simulink model "ultrasonic_sensor"  (R2019a)
settings: Solver=FixedStepAuto  StartTime=0.0  StopTime=inf  RelTol=1e-3  EnableMultiTasking=on
libraries: embdlinuxlib x4, dspswit3 x1
settings Model: SimulationMode=external  Creator=wojna  LastModifiedBy=wojna
settings SolverCC: PositivePriorityOrder=on
settings OptimizationCC: EnhancedBackFolding=on  PassReuseOutputArgsAs=Individual arguments  MaxStackSize=64  OptimizeBlockOrder=speed  DifferentSizesBufferReuse=on  OptimizationCustomize=off
settings DebuggingCC: ParameterTunabilityLossMsg=error
settings HardwareCC: ProdBitPerPointer=32  ProdBitPerSizeT=32  ProdBitPerPtrDiffT=32  ProdLargestAtomicInteger=Long  ProdLargestAtomicFloat=Double  ProdWordSize=32  ProdLongLongMode=on  ProdHWDeviceType=ARM Compatible->ARM Cortex  UseEmbeddedCoderFeatures=off  UseSimulinkCoderFeatures=off
settings SFSimCC: MATLABDynamicMemAlloc=off
settings RTWCC: SystemTargetFile=ert.tlc  HardwareBoard=Raspberry Pi  TLCOptions="-aInlineSetEventsForThisBaseRateFcn=TLC_FALSE -aSuppressMultiTaskScheduler=TLC_FALSE  -aRateBasedStepFcn=0"  TemplateMakefile=ert_default_tmf  RTWVerbose=off  Toolchain=GNU GCC Raspberry Pi  BuildConfiguration=Faster Runs  IncludeHyperlinkInReport=on
settings CodeAppCC: ForceParamTrailComments=on  OperatorAnnotations=on  SimulinkDataObjDesc=on  SFDataObjDesc=on  MangleLength=10  InsertBlockDesc=on
settings ERTTargetCC: SupportNonInlinedSFcns=on  SupportVariableSizeSignals=on  ExtMode=on  ExtModeTransport=2  ExtModeStaticAlloc=on  ExtModeMexFile=ext_xcp  ExtModeMexArgs='192.168.0.101' 0 17725  ExtModeIntrfLevel=Level2 - Open  ERTSrcFileBannerTemplate=codertarget_code_template.cgt  ERTHdrFileBannerTemplate=codertarget_code_template.cgt  ERTDataSrcFileTemplate=codertarget_code_template.cgt  ERTDataHdrFileTemplate=codertarget_code_template.cgt

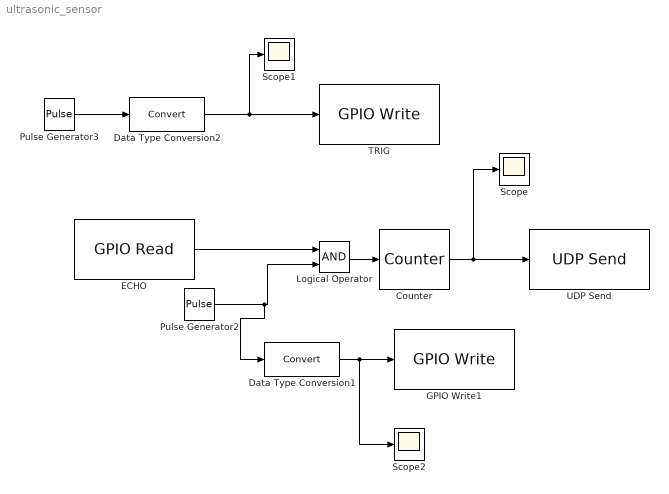
== system ultrasonic_sensor ==
  Counter : dspswit3/Counter  Direction=Up  CountEvent=Rising edge  CounterSize=8 bits  MaxCount=255  InitialCount=0  Output=Count  HitValue=32  ResetInput=off  SamplesPerFrame=1  Ts=1  CntDtype=double  HitDtype=Logical
  Data Type Conversion1 : DataTypeConversion
  Data Type Conversion2 : DataTypeConversion
  ECHO : embdlinuxlib/GPIO Read  board=Pi 3 Model B+  gpio=23  internalResistor=Off  sampleTime=2.5e-05  direction=Input  blockPlatform=Raspberry Pi
      settings: SourceProductName=Simulink Coder Support Package for BeagleBone Blue Hardware  SourceProductBaseCode=SC_BEAGLEBONE_BLUE
  GPIO Write1 : embdlinuxlib/GPIO Write  board=Pi 3 Model B+  gpio=24  direction=Output  blockPlatform=Raspberry Pi
      settings: SourceProductName=Simulink Coder Support Package for BeagleBone Blue Hardware  SourceProductBaseCode=SC_BEAGLEBONE_BLUE
  Logical Operator : Logic  AllPortsSameDT=off  OutDataTypeStr=boolean
  Pulse Generator2 : DiscretePulseGenerator  PulseType=Time based  Amplitude=3  Period=0.00005  PulseWidth=50
  Pulse Generator3 : DiscretePulseGenerator  PulseType=Time based  Amplitude=3  Period=0.1  PulseWidth=0.01
  Scope : Scope
  Scope1 : Scope
  Scope2 : Scope
  TRIG : embdlinuxlib/GPIO Write  board=Pi 3 Model B+  gpio=4  direction=Output  blockPlatform=Raspberry Pi
      settings: SourceProductName=Simulink Coder Support Package for BeagleBone Blue Hardware  SourceProductBaseCode=SC_BEAGLEBONE_BLUE
  UDP Send : embdlinuxlib/UDP Send  remoteURL='255.255.255.255'  remotePort=25000  localURL='255.255.255.255'  localPortSource=Automatically determine  localPort=-1  sampletime=-1  blockPlatform=Raspberry Pi  separateLengthPort=0
      settings: SourceProductName=Simulink Coder Support Package for BeagleBone Blue Hardware  SourceProductBaseCode=SC_BEAGLEBONE_BLUE
  wires:
  Counter/1 -> Scope/1, UDP Send/1
  Pulse Generator2/1 -> Logical Operator/2, Data Type Conversion1/1
  Data Type Conversion1/1 -> Scope2/1, GPIO Write1/1
  ECHO/1 -> Logical Operator/1
  Logical Operator/1 -> Counter/1
  Data Type Conversion2/1 -> Scope1/1, TRIG/1
  Pulse Generator3/1 -> Data Type Conversion2/1
